simulink model "Engine_Airpath_Model"  (R2016b)
settings: Solver=FixedStepAuto  StartTime=0.0  StopTime=inf  FixedStep=EngMdl.tiSimnTiStep_C  RelTol=1e-3  SampleTimeConstraint=STIndependent  EnableMultiTasking=on
undefined symbols (not defined in the file or in its folder): SIM
settings Model: Creator=m01wolf  LastModifiedBy=bunver
settings DataIOCC: SaveFormat=StructureWithTime  SaveOutput=off  DSMLogging=off  VisualizeSimOutput=off  SaveTime=off  StateSaveName=Results  SignalLoggingName=Results
settings OptimizationCC: BlockReduction=off  ConditionallyExecuteInputs=off  LifeSpan=inf
settings DebuggingCC: AllowSymbolicDim=off  SFUnexpectedBacktrackingDiag=warning  SFNoUnconditionalDefaultTransitionDiag=warning  SFExecutionAtInitializationDiag=none
settings ModelReferenceCC: ModelReferenceNumInstancesAllowed=Single  PropagateSignalLabelsOutOfModel=off
settings GRTTargetCC: TargetLangStandard=C89/C90 (ANSI)
settings ConfigComp: CovMetricSettings=dw  CovHtmlReporting=on  CovSaveCumulativeToWorkspaceVar=on  CovSaveSingleToWorkspaceVar=on  CovExternalEMLEnable=off

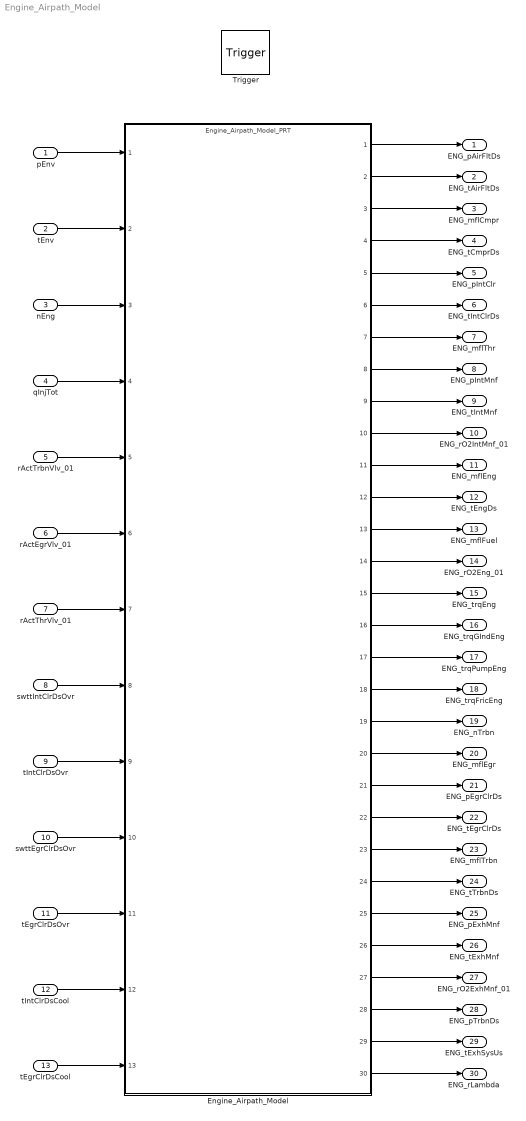
== system Engine_Airpath_Model ==
  pEnv : Inport  OutDataTypeStr=double  PortDimensions=1
  tEnv : Inport  Port=2  OutDataTypeStr=double  PortDimensions=1
  nEng : Inport  Port=3  OutDataTypeStr=double  PortDimensions=1
  qInjTot : Inport  Port=4  OutDataTypeStr=double  PortDimensions=1
  rActTrbnVlv_01 : Inport  Port=5  OutDataTypeStr=double  PortDimensions=1
  rActEgrVlv_01 : Inport  Port=6  OutDataTypeStr=double  PortDimensions=1
  rActThrVlv_01 : Inport  Port=7  OutDataTypeStr=double  PortDimensions=1
  swttIntClrDsOvr : Inport  Port=8  OutDataTypeStr=double  PortDimensions=1
  tIntClrDsOvr : Inport  Port=9  OutDataTypeStr=double  PortDimensions=1
  swttEgrClrDsOvr : Inport  Port=10  OutDataTypeStr=double  PortDimensions=1
  tEgrClrDsOvr : Inport  Port=11  OutDataTypeStr=double  PortDimensions=1
  tIntClrDsCool : Inport  Port=12  OutDataTypeStr=double  PortDimensions=1
  tEgrClrDsCool : Inport  Port=13  OutDataTypeStr=double  PortDimensions=1
  Trigger : TriggerPort  TriggerType=function-call  VariantControl=Variant  SampleTime=SIM.tiSimStepENGPlntAirPath_C  PortDimensions=1  TriggerSignalSampleTime=[0.001,0]
  Engine_Airpath_Model : ModelReference  ModelNameDialog=Engine_Airpath_Model_PRT.slxp  ModelReferenceVersion=1.253  CopyOfModelProtected=on
  ENG_pAirFltDs : Outport
  ENG_tAirFltDs : Outport  Port=2
  ENG_mflCmpr : Outport  Port=3
  ENG_tCmprDs : Outport  Port=4
  ENG_pIntClr : Outport  Port=5
  ENG_tIntClrDs : Outport  Port=6
  ENG_mflThr : Outport  Port=7
  ENG_pIntMnf : Outport  Port=8
  ENG_tIntMnf : Outport  Port=9
  ENG_rO2IntMnf_01 : Outport  Port=10
  ENG_mflEng : Outport  Port=11
  ENG_tEngDs : Outport  Port=12
  ENG_mflFuel : Outport  Port=13
  ENG_rO2Eng_01 : Outport  Port=14
  ENG_trqEng : Outport  Port=15
  ENG_trqGIndEng : Outport  Port=16
  ENG_trqPumpEng : Outport  Port=17
  ENG_trqFricEng : Outport  Port=18
  ENG_nTrbn : Outport  Port=19
  ENG_mflEgr : Outport  Port=20
  ENG_pEgrClrDs : Outport  Port=21
  ENG_tEgrClrDs : Outport  Port=22
  ENG_mflTrbn : Outport  Port=23
  ENG_tTrbnDs : Outport  Port=24
  ENG_pExhMnf : Outport  Port=25
  ENG_tExhMnf : Outport  Port=26
  ENG_rO2ExhMnf_01 : Outport  Port=27
  ENG_pTrbnDs : Outport  Port=28
  ENG_tExhSysUs : Outport  Port=29
  ENG_rLambda : Outport  Port=30
  wires:
  Engine_Airpath_Model/9 -> ENG_tIntMnf/1
  Engine_Airpath_Model/7 -> ENG_mflThr/1
  Engine_Airpath_Model/5 -> ENG_pIntClr/1
  Engine_Airpath_Model/29 -> ENG_tExhSysUs/1
  Engine_Airpath_Model/12 -> ENG_tEngDs/1
  Engine_Airpath_Model/22 -> ENG_tEgrClrDs/1
  Engine_Airpath_Model/20 -> ENG_mflEgr/1
  Engine_Airpath_Model/16 -> ENG_trqGIndEng/1
  Engine_Airpath_Model/30 -> ENG_rLambda/1
  Engine_Airpath_Model/6 -> ENG_tIntClrDs/1
  Engine_Airpath_Model/24 -> ENG_tTrbnDs/1
  Engine_Airpath_Model/3 -> ENG_mflCmpr/1
  Engine_Airpath_Model/14 -> ENG_rO2Eng_01/1
  Engine_Airpath_Model/28 -> ENG_pTrbnDs/1
  Engine_Airpath_Model/4 -> ENG_tCmprDs/1
  Engine_Airpath_Model/10 -> ENG_rO2IntMnf_01/1
  Engine_Airpath_Model/23 -> ENG_mflTrbn/1
  Engine_Airpath_Model/25 -> ENG_pExhMnf/1
  Engine_Airpath_Model/21 -> ENG_pEgrClrDs/1
  Engine_Airpath_Model/27 -> ENG_rO2ExhMnf_01/1
  Engine_Airpath_Model/19 -> ENG_nTrbn/1
  Engine_Airpath_Model/8 -> ENG_pIntMnf/1
  Engine_Airpath_Model/18 -> ENG_trqFricEng/1
  Engine_Airpath_Model/26 -> ENG_tExhMnf/1
  Engine_Airpath_Model/2 -> ENG_tAirFltDs/1
  Engine_Airpath_Model/17 -> ENG_trqPumpEng/1
  Engine_Airpath_Model/15 -> ENG_trqEng/1
  Engine_Airpath_Model/11 -> ENG_mflEng/1
  Engine_Airpath_Model/13 -> ENG_mflFuel/1
  Engine_Airpath_Model/1 -> ENG_pAirFltDs/1
  pEnv/1 -> Engine_Airpath_Model/1
  tEgrClrDsCool/1 -> Engine_Airpath_Model/13
  tEnv/1 -> Engine_Airpath_Model/2
  nEng/1 -> Engine_Airpath_Model/3
  qInjTot/1 -> Engine_Airpath_Model/4
  rActTrbnVlv_01/1 -> Engine_Airpath_Model/5
  rActEgrVlv_01/1 -> Engine_Airpath_Model/6
  rActThrVlv_01/1 -> Engine_Airpath_Model/7
  swttIntClrDsOvr/1 -> Engine_Airpath_Model/8
  tIntClrDsOvr/1 -> Engine_Airpath_Model/9
  swttEgrClrDsOvr/1 -> Engine_Airpath_Model/10
  tEgrClrDsOvr/1 -> Engine_Airpath_Model/11
  tIntClrDsCool/1 -> Engine_Airpath_Model/12
